simulink model "Final_V620140905h5b_fuben1"  (Simulink 7.9)
settings: Solver=FixedStepDiscrete  StartTime=0.0  StopTime=1  FixedStep=Auto  RelTol=1e-3
undefined symbols (not defined in the file or in its folder): Down, Up
libraries: tiiqmathlib x157, idelinklib_common x83, c2833xlib x37, simulink x12, c28xdmclib x12, c280xlib x7, simulink_extras x4, commutil2 x2, idelinklib_tgtpref x1, idelinklib_ticcs x1
(part 1 of 7)
settings Model: Creator=ChenYu  LastModifiedBy=Administrator
settings DataIOCC: SaveOutput=off  SaveTime=off
settings OptimizationCC: OptimizeModelRefInitCode=on  LifeSpan=1
settings HardwareCC: ProdBitPerChar=16  ProdBitPerInt=16  ProdBitPerPointer=16  ProdLargestAtomicInteger=Integer  ProdIntDivRoundTo=Zero  ProdEndianess=LittleEndian  ProdWordSize=16  ProdHWDeviceType=Texas Instruments->C2000
settings RTWCC: SystemTargetFile=idelink_ert.tlc  GenerateMakefile=off  TemplateMakefile=none  Description=IDE Link ERT  ProcessScript=idelink_ert_make_rtw_hook
settings RTWCC: CustomInitializer=|
  | // Make sure the XINTF clock is enabled   cool
  | 	SysCtrlRegs.PCLKCR3.bit.XINTFENCLK = 1;
  | 
  | 	// Configure the GPIO for XINTF with a 16-bit data bus
  | 	// This function is in DSP2833x_Xintf.c
  | 	//InitXintf16Gpio();
  | 
  |     EALLOW;
  |     // All Zones---------------------------------
  |     // Timing for all zones based on XTIMCLK = SYSCLKOUT/2
  |     XintfRegs.XINTCNF2.bit.XTIMCLK = 1;
  |     // Buffer up to 3 writes
  |     XintfRegs.XINTCNF2.bit.WRBUFF = 3;
  |     // XCLKOUT is enabled
  |     XintfRegs.XINTCNF2.bit.CLKOFF = 0;
  |     // XCLKOUT = XTIMCLK/2
  |     XintfRegs.XINTCNF2.bit.CLKMODE = 1;
  | 
  |     // Zone 7------------------------------------
  |     // When using ready, ACTIVE must be 1 or greater
  |     // Lead must always be 1 or greater
  |     // Zone write timing
  |     XintfRegs.XTIMING7.bit.XWRLEAD = 3;//3*2*2*SYSCLKOUT
  |     XintfRegs.XTIMING7.bit.XWRACTIVE = 7; //(7+1)*2*2*SYSCLKOUT
  |     XintfRegs.XTIMING7.bit.XWRTRAIL = 3;
  |     // Zone read timing
  |     XintfRegs.XTIMING7.bit.XRDLEAD = 3;
  |     XintfRegs.XTIMING7.bit.XRDACTIVE = 7;
  |     XintfRegs.XTIMING7.bit.XRDTRAIL = 3;
  | 
  |     // double all Zone read/write lead/active/trail timing
  |     XintfRegs.XTIMING7.bit.X2TIMING = 1;
  | 
  |     // Zone will not sample XREADY signal
  |     XintfRegs.XTIMING7.bit.USEREADY = 0;
  |     XintfRegs.XTIMING7.bit.READYMODE = 0;
  | 
  |     // Size must be either:
  |     // 0,1 = x32 or
  |     // 1,1 = x16 other values are reserved
  |     XintfRegs.XTIMING7.bit.XSIZE = 3;
  | 
  |     EDIS;
  | 
  |    //Force a pipeline flush to ensure that the write to
  |    //the last register configured occurs before returning.
  |    asm(" RPT #7 || NOP");
settings CodeAppCC: IgnoreCustomStorageClasses=off
settings ERTFactory: TargetFcnLib=ansi_tfl_table_tmw.mat  CodeReplacementLibrary=ANSI_C  UtilityFuncGeneration=Auto  ERTMultiwordTypeDef=System defined  CodeExecutionProfiling=off  ERTMultiwordLength=256  MultiwordLength=2048  GenerateFullHeader=on  GenerateSampleERTMain=off  GenerateTestInterfaces=off  IsPILTarget=off  ModelReferenceCompliant=on  ParMdlRefBuildCompliant=off  CompOptLevelCompliant=off  ConcurrentExecutionCompliant=on  IncludeMdlTerminateFcn=on  GeneratePreprocessorConditionals=Disable all  CombineOutputUpdateFcns=on  CombineSignalStateStructs=off  SuppressErrorStatus=off  ERTFirstTimeCompliant=on  IncludeFileDelimiter=Auto  ERTCustomFileBanners=on  SupportAbsoluteTime=on  LogVarNameModifier=rt_  MatFileLogging=off  MultiInstanceERTCode=off  SupportNonFinite=on  SupportComplex=on  PurelyIntegerCode=off  SupportContinuousTime=off  SupportNonInlinedSFcns=off  SupportVariableSizeSignals=off  EnableShiftOperators=on  ParenthesesLevel=Nominal  PortableWordSizes=off  ModelStepFunctionPrototypeControlCompliant=on  CPPClassGenCompliant=off  AutosarCompliant=off  GRTInterface=off  GenerateErtSFunction=off  CreateSILPILBlock=None  CodeExecutionProfileVariable=executionProfile  CodeProfilingSaveOptions=SummaryOnly  GenerateASAP2=off  ExtMode=off  ExtModeTransport=0  ExtModeStaticAlloc=off  ExtModeStaticAllocSize=1000000  ExtModeTesting=off  ExtModeMexFile=TIC2000ExternalModeOpen  ExtModeIntrfLevel=Level2 - Open  InlinedParameterPlacement=Hierarchical  TargetOS=BareBoardExample  MultiInstanceErrorCode=Error  RateGroupingCode=on  RootIOFormat=Individual arguments  RTWCAPISignals=off  RTWCAPIParams=off  RTWCAPIStates=off  RTWCAPIRootIO=off  ERTSrcFileBannerTemplate=ert_code_template.cgt  ERTHdrFileBannerTemplate=ert_code_template.cgt  ERTDataSrcFileTemplate=ert_code_template.cgt  ERTDataHdrFileTemplate=ert_code_template.cgt  ERTCustomFileTemplate=example_file_process.tlc  CoverageDialogOpen=off  EnableDataOwnership=off  SignalDisplayLevel=10  ParamTuneLevel=10  GlobalDataDefinition=Auto  DataDefinitionFile=global.c  GlobalDataReference=Auto  ERTFilePackagingFormat=Modular  DataReferenceFile=global.h  PreserveExpressionOrder=off  PreserveIfCondition=off  ConvertIfToSwitch=off  PreserveExternInFcnDecls=on  SuppressUnreachableDefaultCases=off  EnableUserReplacementTypes=off  MemSecPackage=--- None ---  MemSecDataConstants=Default  MemSecDataIO=Default  MemSecDataInternal=Default  MemSecDataParameters=Default  MemSecFuncInitTerm=Default  MemSecFuncExecute=Default  MemSecFuncSharedUtil=Default  CodeProfilingInstrumentation=off  AdaptorName=Texas Instruments Code Composer Studio  exportIDEObj=on  ideObjName=IDE_Obj  oldideObjName=IDE_Obj  ideObjTimeout=10  oldideObjTimeout=10  ideObjBuildTimeout=1000  oldideObjBuildTimeout=1000  TargetPrefTimeStamp=30-Jun-2014 19:43:40  ProfileGenCode=on  profileBy=Tasks  ProfileNumSamples=100  InlineDSPBlks=off  projectOptions=Custom  debugCompilerOptions="-g -D\"_DEBUG\""  releaseCompilerOptions=-o2  getCompilerOptions=off  resetCompilerOptions=off  getLinkerOptions=off  resetLinkerOptions=off  systemStackSize=512  systemHeapSize=512  buildFormat=Project  buildAction=Build  overrunNotificationMethod=None  overrunNotificationFcn=myfunction  oldoverrunNotificationFcn=myfunction  configurePIL=off  configPILBlockAction=Create_PIL_block_build_and_download  DiagnosticActions=warning

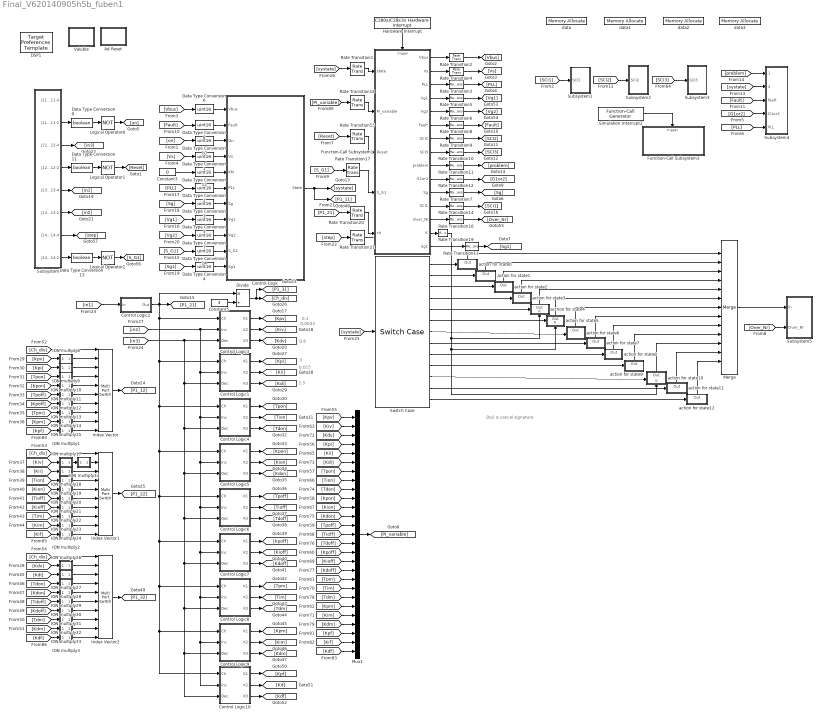
== system Final_V620140905h5b_fuben1 ==
  note: Do2 is cancel signature
  note: 3
  note: 0.015
  note: 2.5
  note: 0.1
  note: 0.0033
  note: 0.6
  Ad Reset : Subsystem
  Constant3 : Constant  Value=0  OutDataTypeStr=uint16
  Constant5 : Constant  Value=3  OutDataTypeStr=uint16
  Control Logic : Stateflow chart  TreatAsAtomicUnit=on
  Control Logic1 : Stateflow chart  TreatAsAtomicUnit=on
  Control Logic10 : Stateflow chart  TreatAsAtomicUnit=on
  Control Logic2 : Stateflow chart  TreatAsAtomicUnit=on
  Control Logic3 : Stateflow chart  TreatAsAtomicUnit=on
  Control Logic4 : Stateflow chart  TreatAsAtomicUnit=on
  Control Logic5 : Stateflow chart  TreatAsAtomicUnit=on
  Control Logic6 : Stateflow chart  TreatAsAtomicUnit=on
  Control Logic7 : Stateflow chart  TreatAsAtomicUnit=on
  Control Logic8 : Stateflow chart  TreatAsAtomicUnit=on
  Control Logic9 : Stateflow chart  TreatAsAtomicUnit=on
  DSP1 : idelinklib_tgtpref/Target Preferences Template  Tag=ccslinktgtpref  library=off
  Data Type Conversion{1..8,10,12,14} (11 alike) : DataTypeConversion  OutDataTypeStr=uint16
  Data Type Conversion11 : DataTypeConversion  OutDataTypeStr=boolean
  Data Type Conversion13 : DataTypeConversion  OutDataTypeStr=boolean
  Data Type Conversion9 : DataTypeConversion  OutDataTypeStr=boolean
  Divide : Product  Inputs=*/
  Function-Call Subsystem1 : Subsystem  TreatAsAtomicUnit=on
  Function-Call Subsystem3 : Subsystem  TreatAsAtomicUnit=on
  Hardware Interrupt : idelinklib_ticcs/C280x//C28x3x Hardware Interrupt  Priority=3  irqnumbers=[3]  pienumbers=[4]  irqpriorities=[30]  irqpreempts=[0]  showinput=off  dspchiptype=C280X
  ION multiply1 : Subsystem  mask{x=1}
      mask prompts: x "gain"
  ION multiply10 : Subsystem  mask{x=10}
      mask prompts: x "gain"
  ION multiply11 : Subsystem  mask{x=100}
      mask prompts: x "gain"
  ION multiply12 : Subsystem  mask{x=10}
      mask prompts: x "gain"
  ION multiply13 : Subsystem  mask{x=100}
      mask prompts: x "gain"
  ION multiply14 : Subsystem  mask{x=10}
      mask prompts: x "gain"
  ION multiply15 : Subsystem  mask{x=100}
      mask prompts: x "gain"
  ION multiply17 : Subsystem  mask{x=1000}
      mask prompts: x "gain"
  ION multiply18 : Subsystem  mask{x=1000}
      mask prompts: x "gain"
  ION multiply19 : Subsystem  mask{x=10}
      mask prompts: x "gain"
  ION multiply2 : Subsystem  mask{x=10}
      mask prompts: x "gain"
  ION multiply20 : Subsystem  mask{x=1000}
      mask prompts: x "gain"
  ION multiply21 : Subsystem  mask{x=10}
      mask prompts: x "gain"
  ION multiply22 : Subsystem  mask{x=100}
      mask prompts: x "gain"
  ION multiply23 : Subsystem  mask{x=10}
      mask prompts: x "gain"
  ION multiply24 : Subsystem  mask{x=1000}
      mask prompts: x "gain"
  ION multiply26 : Subsystem  mask{x=10}
      mask prompts: x "gain"
  ION multiply27 : Subsystem  mask{x=10}
      mask prompts: x "gain"
  ION multiply28 : Subsystem  mask{x=10}
      mask prompts: x "gain"
  ION multiply29 : Subsystem  mask{x=10}
      mask prompts: x "gain"
  ION multiply3 : Subsystem  mask{x=10}
      mask prompts: x "gain"
  ION multiply30 : Subsystem  mask{x=10}
      mask prompts: x "gain"
  ION multiply31 : Subsystem  mask{x=10}
      mask prompts: x "gain"
  ION multiply32 : Subsystem  mask{x=10}
      mask prompts: x "gain"
  ION multiply33 : Subsystem  mask{x=10}
      mask prompts: x "gain"
  ION multiply34 : Subsystem  mask{x=10}
      mask prompts: x "gain"
  ION multiply8 : Subsystem  mask{x=100}
      mask prompts: x "gain"
  ION multiply9 : Subsystem  mask{x=10}
      mask prompts: x "gain"
  Index Vector : MultiPortSwitch  DataPortOrder=Zero-based contiguous  Inputs=9  zeroidx=on
  Index Vector1 : MultiPortSwitch  DataPortOrder=Zero-based contiguous  Inputs=9  zeroidx=on
  Index Vector2 : MultiPortSwitch  DataPortOrder=Zero-based contiguous  Inputs=9  zeroidx=on
  Logical Operator1 : Logic  Operator=NOT  AllPortsSameDT=off  OutDataTypeStr=boolean
  Logical Operator2 : Logic  Operator=NOT  AllPortsSameDT=off  OutDataTypeStr=boolean
  Logical Operator6 : Logic  Operator=NOT  AllPortsSameDT=off  OutDataTypeStr=boolean
  Merge : Merge  Inputs=13
  Mux1 : Mux  Inputs=27
  Rate Transition{1..21} (21 alike) : RateTransition  Integrity=off
  Simulation Interrupt2 : simulink/Ports & Subsystems/Function-Call Generator  sample_time=0.05  numberOfIterations=1
  Subsystem : Subsystem
  Subsystem1 : Subsystem
  Subsystem2 : Subsystem
  Subsystem3 : Subsystem
  Subsystem4 : Subsystem
  Subsystem5 : Subsystem
  Switch Case : SwitchCase  CaseConditions={0,1,2,3,4,5,6,7,8,9,10,11,12}  ShowDefaultCase=off
  Valuble : Subsystem
  action for state0 : Subsystem  TreatAsAtomicUnit=on
  action for state1 : Subsystem  TreatAsAtomicUnit=on
  action for state10 : Subsystem  TreatAsAtomicUnit=on
  action for state11 : Subsystem  TreatAsAtomicUnit=on
  action for state12 : Subsystem  TreatAsAtomicUnit=on
  action for state2 : Subsystem  TreatAsAtomicUnit=on
  action for state3 : Subsystem  TreatAsAtomicUnit=on
  action for state5 : Subsystem  TreatAsAtomicUnit=on
  action for state6 : Subsystem  TreatAsAtomicUnit=on
  action for state7 : Subsystem  TreatAsAtomicUnit=on
  action for state8 : Subsystem  TreatAsAtomicUnit=on
  action for state9 : Subsystem  TreatAsAtomicUnit=on
  actrion for state4 : Subsystem  TreatAsAtomicUnit=on
  data : idelinklib_common/Memory Allocate  variableName=data  alignThisVariable=off  memoryAlignmentBoundary=4  dataType=int16  specifyQualifier=off  typeQualifier=volatile  dataDimension=8  specifyMemorySection=off  memorySection=mySEC1  bindMemorySection=on  sectionStartAddress=hex2dec('8000')  initializeMemory=on  initialValue=0
  data1 : idelinklib_common/Memory Allocate  variableName=data1  alignThisVariable=off  memoryAlignmentBoundary=4  dataType=int16  specifyQualifier=off  typeQualifier=volatile  dataDimension=8  specifyMemorySection=off  memorySection=mySEC1  bindMemorySection=on  sectionStartAddress=hex2dec('8000')  initializeMemory=on  initialValue=0
  data2 : idelinklib_common/Memory Allocate  variableName=data2  alignThisVariable=off  memoryAlignmentBoundary=4  dataType=int16  specifyQualifier=off  typeQualifier=volatile  dataDimension=8  specifyMemorySection=off  memorySection=mySEC1  bindMemorySection=on  sectionStartAddress=hex2dec('8000')  initializeMemory=on  initialValue=0
  data3 : idelinklib_common/Memory Allocate  variableName=data3  alignThisVariable=off  memoryAlignmentBoundary=4  dataType=int16  specifyQualifier=off  typeQualifier=volatile  dataDimension=8  specifyMemorySection=off  memorySection=mySEC1  bindMemorySection=on  sectionStartAddress=hex2dec('8000')  initializeMemory=on  initialValue=0
  wires:
  Switch Case/1 -> action for state0/Action
  Switch Case/2 -> action for state1/Action
  Switch Case/3 -> action for state2/Action
  Switch Case/4 -> action for state3/Action
  Switch Case/5 -> actrion for state4/Action
  Switch Case/6 -> action for state5/Action
  [Fault] -> Data Type Conversion8/1
  [Vbus] -> Data Type Conversion6/1
  [on] -> Data Type Conversion10/1
  Subsystem/4(J12-1&J12-2) -> Data Type Conversion11/1
  Control Logic/1(State) -> [systate], [P1_11]
  Data Type Conversion6/1 -> Control Logic/1(Vbus)
  [Vs] -> Data Type Conversion1/1
  Constant3/1 -> Data Type Conversion12/1
  Data Type Conversion1/1 -> Control Logic/4(Vs)
  Hardware Interrupt/1 -> Function-Call Subsystem1/Trigger
  Data Type Conversion2/1 -> Control Logic/6(PLL)
  [PLL] -> Data Type Conversion2/1
  [Sg] -> Data Type Conversion3/1
  Data Type Conversion3/1 -> Control Logic/7(Sg)
  [Vg1] -> Data Type Conversion5/1
  [Vg2] -> Data Type Conversion7/1
  Switch Case/7 -> action for state6/Action
  Switch Case/8 -> action for state7/Action
  Data Type Conversion8/1 -> Control Logic/2(Fault)
  Simulation Interrupt2/1 -> Function-Call Subsystem3/Trigger
  [SCI3] -> Subsystem3/1(SCI3)
  [SCI2] -> Subsystem2/1(SCI2)
  [systate] -> Subsystem4/2(systate)
  [problem] -> Subsystem4/1(problem)
  [Fault] -> Subsystem4/3(fault)
  Data Type Conversion7/1 -> Control Logic/9(Vg2)
  [G1or2] -> Subsystem4/4(G1or2)
  [PLL] -> Subsystem4/5(PLL)
  Switch Case/9 -> action for state8/Action
  Switch Case/10 -> action for state9/Action
  Switch Case/11 -> action for state10/Action
  Switch Case/12 -> action for state11/Action
  Data Type Conversion5/1 -> Control Logic/8(Vg1)
  Switch Case/13 -> action for state12/Action
  Function-Call Subsystem1/1(Vbus) -> Rate Transition2/1
  Function-Call Subsystem1/2(Vs) -> Rate Transition4/1
  Function-Call Subsystem1/3(PLL) -> Rate Transition3/1
  Rate Transition2/1 -> [Vbus]
  Rate Transition4/1 -> [Vs]
  Rate Transition3/1 -> [PLL]
  Function-Call Subsystem1/4(Vg1) -> Rate Transition5/1
  Function-Call Subsystem1/5(Vg2) -> Rate Transition6/1
  Function-Call Subsystem1/6(Fault) -> Rate Transition8/1
  Rate Transition8/1 -> [Fault]
  Function-Call Subsystem1/7(SCI2) -> Rate Transition9/1
  Rate Transition9/1 -> [SCI2]
  Function-Call Subsystem1/8(SCI3) -> Rate Transition10/1
  Rate Transition10/1 -> [SCI3]
  Rate Transition11/1 -> [problem]
  Function-Call Subsystem1/9(problem) -> Rate Transition11/1
  Rate Transition5/1 -> [Vg1]
  Rate Transition6/1 -> [Vg2]
  Function-Call Subsystem1/10(G1or2) -> Rate Transition12/1
  Rate Transition12/1 -> [G1or2]
  Data Type Conversion10/1 -> Control Logic/3(On)
  Data Type Conversion9/1 -> Logical Operator6/1
  Subsystem/2(J11-1&J11-2) -> Data Type Conversion9/1
  Logical Operator6/1 -> [on]
  [systate] -> Switch Case/1
  [systate] -> Rate Transition1/1
  Rate Transition1/1 -> Function-Call Subsystem1/1(state)
  Data Type Conversion12/1 -> Control Logic/5(KM)
  Control Logic2/1(Out) -> [P1_21], Control Logic3/1(Ch), Control Logic4/1(Ch), Control Logic5/1(Ch), Control Logic6/1(Ch), Control Logic7/1(Ch), Control Logic8/1(Ch), Control Logic9/1(Ch), Control Logic10/1(Ch), Control Logic1/1(Ch), Divide/1
  Subsystem/5(J13-3&J13-4) -> [in1]
  [in1] -> Control Logic2/1(In)
  Subsystem/6(J13-1&J13-2) -> [in2]
  [in2] -> Control Logic3/2(Inc), Control Logic1/2(Inc), Control Logic4/2(Inc), Control Logic5/2(Inc), Control Logic6/2(Inc), Control Logic7/2(Inc), Control Logic8/2(Inc), Control Logic9/2(Inc), Control Logic10/2(Inc)
  [in3] -> Control Logic3/3(Dec), Control Logic1/3(Dec), Control Logic4/3(Dec), Control Logic5/3(Dec), Control Logic6/3(Dec), Control Logic7/3(Dec), Control Logic8/3(Dec), Control Logic9/3(Dec), Control Logic10/3(Dec)
  Subsystem/3(J12-3&J12-4) -> [in3]
  Index Vector/1 -> [P1_12]
  Divide/1 -> [P1_31], [Ch_dis]
  Constant5/1 -> Divide/2
  Control Logic3/1(K1) -> [Kpv]
  Control Logic3/2(K2) -> [Kiv]
  Control Logic3/3(K3) -> [Kdv]
  Control Logic1/1(K1) -> [Kpi]
  Control Logic1/2(K2) -> [Kii]
  Control Logic1/3(K3) -> [Kdi]
  Control Logic4/1(K1) -> [Tpon]
  Control Logic4/2(K2) -> [Tion]
  Control Logic4/3(K3) -> [Tdon]
  Control Logic5/1(K1) -> [Kpon]
  Control Logic5/2(K2) -> [Kion]
  Control Logic5/3(K3) -> [Kdon]
  Control Logic6/1(K1) -> [Tpoff]
  Control Logic6/2(K2) -> [Tioff]
  Control Logic6/3(K3) -> [Tdoff]
  Control Logic7/1(K1) -> [Kpoff]
  Control Logic7/2(K2) -> [Kioff]
  Control Logic7/3(K3) -> [Kdoff]
  Control Logic8/1(K1) -> [Tpm]
  Control Logic8/2(K2) -> [Tim]
  Control Logic8/3(K3) -> [Tdm]
  Control Logic9/1(K1) -> [Kpm]
  Control Logic9/2(K2) -> [Kim]
  Control Logic9/3(K3) -> [Kdm]
  [Kpv] -> ION multiply8/1(x)
  [Tpoff] -> ION multiply12/1(x)
  [Kpoff] -> ION multiply13/1(x)
  [Tpm] -> ION multiply14/1(x)
  [Kpm] -> ION multiply15/1(x)
  [Kpi] -> ION multiply9/1(x)
  [Tpon] -> ION multiply10/1(x)
  [Kpon] -> ION multiply11/1(x)
  [Kiv] -> ION multiply17/1(x)
  [Tioff] -> ION multiply21/1(x)
  [Kioff] -> ION multiply22/1(x)
  [Tim] -> ION multiply23/1(x)
  [Kim] -> ION multiply24/1(x)
  [Kii] -> ION multiply18/1(x)
  [Tion] -> ION multiply19/1(x)
  [Kion] -> ION multiply20/1(x)
  Index Vector1/1 -> [P1_22]
  [Kdv] -> ION multiply26/1(x)
  [Tdoff] -> ION multiply30/1(x)
  [Kdoff] -> ION multiply31/1(x)
  [Tdm] -> ION multiply32/1(x)
  [Kdm] -> ION multiply33/1(x)
  [Kdi] -> ION multiply27/1(x)
  [Tdon] -> ION multiply28/1(x)
  [Kdon] -> ION multiply29/1(x)
  Index Vector2/1 -> [P1_32]
  [Ch_dis] -> Index Vector/1
  [Ch_dis] -> Index Vector1/1
  [Ch_dis] -> Index Vector2/1
  ION multiply8/1(Kx) -> Index Vector/2
  ION multiply9/1(Kx) -> Index Vector/3
  ION multiply10/1(Kx) -> Index Vector/4
  ION multiply11/1(Kx) -> Index Vector/5
  ION multiply12/1(Kx) -> Index Vector/6
  ION multiply13/1(Kx) -> Index Vector/7
  ION multiply14/1(Kx) -> Index Vector/8
  ION multiply15/1(Kx) -> Index Vector/9
  ION multiply17/1(Kx) -> ION multiply34/1(x)
  ION multiply18/1(Kx) -> Index Vector1/3
  ION multiply19/1(Kx) -> Index Vector1/4
  ION multiply20/1(Kx) -> Index Vector1/5
  ION multiply21/1(Kx) -> Index Vector1/6
  ION multiply22/1(Kx) -> Index Vector1/7
  ION multiply23/1(Kx) -> Index Vector1/8
  ION multiply24/1(Kx) -> Index Vector1/9
  ION multiply26/1(Kx) -> Index Vector2/2
  ION multiply27/1(Kx) -> Index Vector2/3
  ION multiply28/1(Kx) -> Index Vector2/4
  ION multiply29/1(Kx) -> Index Vector2/5
  ION multiply30/1(Kx) -> Index Vector2/6
  ION multiply31/1(Kx) -> Index Vector2/7
  ION multiply32/1(Kx) -> Index Vector2/8
  ION multiply33/1(Kx) -> Index Vector2/9
  ION multiply34/1(Kx) -> Index Vector1/2
  [Kpv] -> Mux1/1
  [Kiv] -> Mux1/2
  [Kdv] -> Mux1/3
  [Kpi] -> Mux1/4
  [Kii] -> Mux1/5
  [Kdi] -> Mux1/6
  [Tpon] -> Mux1/7
  [Tion] -> Mux1/8
  [Tdon] -> Mux1/9
  [Kpon] -> Mux1/10
  [Kion] -> Mux1/11
  [Kdon] -> Mux1/12
  [Tpoff] -> Mux1/13
  [Tdoff] -> Mux1/15
  [Kpoff] -> Mux1/16
  [Tioff] -> Mux1/14
  [Kioff] -> Mux1/17
  [Kdoff] -> Mux1/18
  [Tpm] -> Mux1/19
  [Tim] -> Mux1/20
  [Tdm] -> Mux1/21
  [Kpm] -> Mux1/22
  [Kim] -> Mux1/23
  [Kdm] -> Mux1/24
  Mux1/1 -> [PI_variable]
  [PI_variable] -> Rate Transition18/1
  Rate Transition18/1 -> Function-Call Subsystem1/2(PI_variable)
  [Kpf] -> Mux1/25
  [Kif] -> Mux1/26
  [Kdf] -> Mux1/27
  Control Logic10/1(K1) -> [Kpf]
  Control Logic10/2(K2) -> [Kif]
  Control Logic10/3(K3) -> [Kdf]
  [Kpf] -> ION multiply1/1(x)
  [Kif] -> ION multiply2/1(x)
  [Kdf] -> ION multiply3/1(x)
  ION multiply1/1(Kx) -> Index Vector/10
  ION multiply2/1(Kx) -> Index Vector1/10
  ION multiply3/1(Kx) -> Index Vector2/10
  Function-Call Subsystem1/11(Sg) -> Rate Transition7/1
  Rate Transition7/1 -> [Sg]
  Function-Call Subsystem1/12(SCI1) -> Rate Transition14/1
  Rate Transition14/1 -> [SCI1]
  [SCI1] -> Subsystem1/1(SCI1)
  Data Type Conversion11/1 -> Logical Operator1/1
  Logical Operator1/1 -> [Reset]
  [Reset] -> Rate Transition15/1
  Rate Transition15/1 -> Function-Call Subsystem1/3(Reset)
  Function-Call Subsystem1/13(Over_Nr) -> Rate Transition16/1
  Rate Transition16/1 -> [Over_Nr]
  Merge/1 -> Subsystem5/1(In)
  action for state0/1(Out) -> Merge/1
  action for state1/1(Out) -> Merge/2
  action for state2/1(Out) -> Merge/3
  action for state3/1(Out) -> Merge/4
  actrion for state4/1(Out) -> Merge/5
  action for state5/1(Out) -> Merge/6
  action for state6/1(Out) -> Merge/7
  action for state7/1(Out) -> Merge/8
  action for state8/1(Out) -> Merge/9
  action for state9/1(Out) -> Merge/10
  action for state10/1(Out) -> Merge/11
  action for state11/1(Out) -> Merge/12
  action for state12/1(Out) -> Merge/13
  [Over_Nr] -> Subsystem5/2(Over_Nr)
  Subsystem/8(J14-1&J14-2) -> Data Type Conversion13/1
  Rate Transition17/1 -> Function-Call Subsystem1/4(S_G1)
  [S_G1] -> Rate Transition17/1
  Data Type Conversion13/1 -> Logical Operator2/1
  Logical Operator2/1 -> [S_G1]
  Function-Call Subsystem1/14(K) -> Rate Transition19/1
  Rate Transition19/1 -> actrion for state4/1(K), action for state5/1(K), action for state10/1(K)
  Data Type Conversion14/1 -> Control Logic/10(S_G1)
  [S_G1] -> Data Type Conversion14/1
  [P1_21] -> Rate Transition20/1
  Rate Transition20/1 -> Function-Call Subsystem1/5(ch)
  Function-Call Subsystem1/15(Sg1) -> Rate Transition13/1
  Rate Transition13/1 -> [Sg1]
  [Sg1] -> Data Type Conversion4/1
  Data Type Conversion4/1 -> Control Logic/11(Sg1)
  Subsystem/7(J14-3&J14-4) -> [step]
  [step] -> Rate Transition21/1
  Rate Transition21/1 -> ?

== system Final_V620140905h5b_fuben1/Ad Reset ==
  Ad Reset : c2833xlib/Digital Output  Priority=1  GPIO_Number=GPIO56~GPIO63  GPIO_Bit0=off  GPIO_BIT0_Toggle=off  GPIO_Bit1=off  GPIO_BIT1_Toggle=off  GPIO_Bit2=off  GPIO_BIT2_Toggle=off  GPIO_Bit3=off  GPIO_BIT3_Toggle=off  GPIO_Bit4=off  GPIO_BIT4_Toggle=off  GPIO_Bit5=on  GPIO_BIT5_Toggle=off  GPIO_Bit6=off  GPIO_BIT6_Toggle=off  GPIO_Bit7=off  GPIO_BIT7_Toggle=off
  Ad1 start : c2833xlib/Digital Output  Priority=2  GPIO_Number=GPIO56~GPIO63  GPIO_Bit0=off  GPIO_BIT0_Toggle=off  GPIO_Bit1=on  GPIO_BIT1_Toggle=off  GPIO_Bit2=off  GPIO_BIT2_Toggle=off  GPIO_Bit3=off  GPIO_BIT3_Toggle=off  GPIO_Bit4=off  GPIO_BIT4_Toggle=off  GPIO_Bit5=off  GPIO_BIT5_Toggle=off  GPIO_Bit6=off  GPIO_BIT6_Toggle=off  GPIO_Bit7=off  GPIO_BIT7_Toggle=off
  Ad2 start1 : c2833xlib/Digital Output  Priority=2  GPIO_Number=GPIO56~GPIO63  GPIO_Bit0=off  GPIO_BIT0_Toggle=off  GPIO_Bit1=off  GPIO_BIT1_Toggle=off  GPIO_Bit2=on  GPIO_BIT2_Toggle=off  GPIO_Bit3=off  GPIO_BIT3_Toggle=off  GPIO_Bit4=off  GPIO_BIT4_Toggle=off  GPIO_Bit5=off  GPIO_BIT5_Toggle=off  GPIO_Bit6=off  GPIO_BIT6_Toggle=off  GPIO_Bit7=off  GPIO_BIT7_Toggle=off
  Add1 : Sum  Inputs=+-
  Constant : Constant  Value=0
  Constant1 : Constant  Value=0
  Step : Step  Time=0
  Step1 : Step  Time=0.01
  wires:
  Step/1 -> Add1/1
  Step1/1 -> Add1/2
  Add1/1 -> Ad Reset/1
  Constant/1 -> Ad1 start/1
  Constant1/1 -> Ad2 start1/1
